simulink model "pwm"  (R2021a)
settings: Solver=VariableStepAuto  StartTime=0.0  StopTime=10.0  RelTol=1e-3
settings Model: Creator=simut  LastModifiedBy=simut

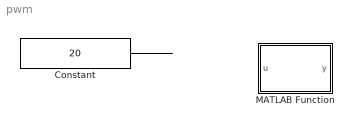
== system pwm ==
  Constant : Constant  Value=20
  MATLAB Function : MATLAB Function  TreatAsAtomicUnit=on
  wires:
  Constant/1 -> ?

== matlab function pwm/MATLAB Function ==
  data: u input; y output
function y = thrust_to_PWM(u)

c0 = 32602.483139300428;
c1 = 1757.9542617659604;
y = c0 + c1*u;
